simulink subsystem "battery_InputNoise"  (R2022a)
settings: Solver=VariableStepAuto  StartTime=0.0  StopTime=10.0  RelTol=1e-3
values from neighbouring files (symbols this model uses):
  C_des = SIM.OutputMatrix    [RunSimulink.m]
  C_m = C_des(P.cell_voltage,:)    [RunSimulink.m]
  K = -diag(diag_vec)    [getLCParam.m]
  M_cross = LC_param.M_cross    [RunSimulink.m]    (also in getLCParam.m = V*S_cross*U')
  SV_IC = SIM.x_0_FOM    [RunSimulink.m]
  U_NV_NT = LC_param.U_NV_NT    [RunSimulink.m]    (also in getLCParam.m = U_null*V_null')
undefined symbols (not defined in the file or in its folder): AN, CA, CONS, EL, FLAG, N, P, PROPS, SEP, SIM, tc
libraries: simulink x2
settings Model: Creator=tyevans  LastModifiedBy=tyevans

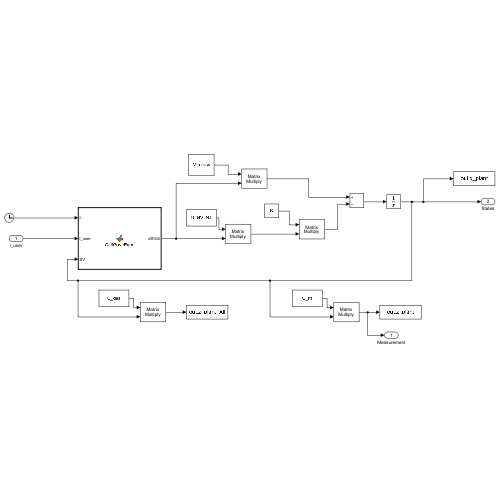
[thumbnail: Simulink's stored preview of the top-level diagram]
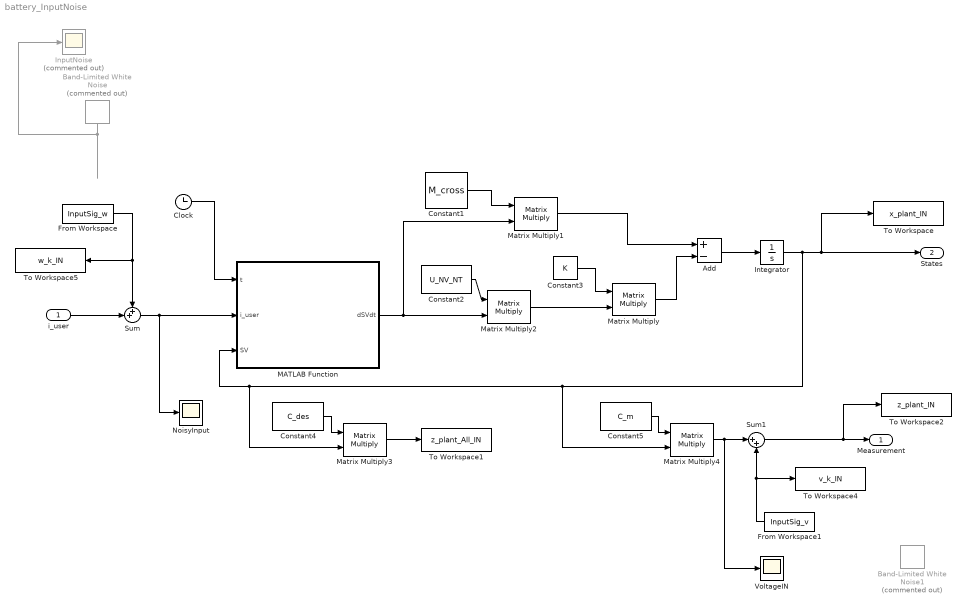
== system battery_InputNoise ==
  i_user : Inport
  Add : Sum  Inputs=+-
  Band-Limited White Noise : simulink/Sources/Band-Limited White Noise  Commented=on  Cov=pow_Qi  Ts=tc  seed=[100]  VectorParams1D=off
  Band-Limited White Noise1 : simulink/Sources/Band-Limited White Noise  Commented=on  Cov=pow_R  Ts=tc  seed=[23341]  VectorParams1D=off
  Clock : Clock
  Constant1 : Constant  Value=M_cross  VectorParams1D=off
  Constant2 : Constant  Value=U_NV_NT  VectorParams1D=off
  Constant3 : Constant  Value=K  VectorParams1D=off
  Constant4 : Constant  Value=C_des  VectorParams1D=off
  Constant5 : Constant  Value=C_m  VectorParams1D=off
  From Workspace : FromWorkspace  VariableName=InputSig_w  OutputAfterFinalValue=Holding final value
  From Workspace1 : FromWorkspace  VariableName=InputSig_v  OutputAfterFinalValue=Holding final value
  InputNoise : Scope  Commented=on
  Integrator : Integrator  InitialCondition=SV_IC
  MATLAB Function : MATLAB Function  TreatAsAtomicUnit=on
  Matrix Multiply{,1..4} (5 alike) : Product  Multiplication=Matrix(*)
  NoisyInput : Scope
  Sum : Sum  Inputs=++|
  Sum1 : Sum  Inputs=|++
  To Workspace : ToWorkspace  VariableName=x_plant_IN  SaveFormat=Structure With Time  SampleTime=-1
  To Workspace1 : ToWorkspace  VariableName=z_plant_All_IN  SaveFormat=Structure With Time  SampleTime=-1
  To Workspace2 : ToWorkspace  VariableName=z_plant_IN  SaveFormat=Structure With Time  SampleTime=-1
  To Workspace4 : ToWorkspace  VariableName=v_k_IN  SaveFormat=Structure With Time  SampleTime=-1
  To Workspace5 : ToWorkspace  VariableName=w_k_IN  SaveFormat=Structure With Time  SampleTime=-1
      settings: Save2DSignal=2-D array (concatenate along first dimension)
  VoltageIN : Scope
  Measurement : Outport
  States : Outport  Port=2
  wires:
  Constant2/1 -> Matrix Multiply2/1
  Matrix Multiply/1 -> Add/2
  Matrix Multiply1/1 -> Add/1
  Clock/1 -> MATLAB Function/1(t)
  Constant3/1 -> Matrix Multiply/1
  Constant4/1 -> Matrix Multiply3/1
  Matrix Multiply3/1 -> To Workspace1/1
  Constant1/1 -> Matrix Multiply1/1
  Add/1 -> Integrator/1
  MATLAB Function/1(dSVdt) -> Matrix Multiply2/2, Matrix Multiply1/2
  Matrix Multiply2/1 -> Matrix Multiply/2
  Constant5/1 -> Matrix Multiply4/1
  Integrator/1 -> States/1, To Workspace/1, Matrix Multiply4/2, Matrix Multiply3/2, MATLAB Function/3(SV)
  From Workspace1/1 -> Sum1/2, To Workspace4/1
  Matrix Multiply4/1 -> Sum1/1, VoltageIN/1
  Sum1/1 -> To Workspace2/1, Measurement/1
  i_user/1 -> Sum/2
  Sum/1 -> MATLAB Function/2(i_user), NoisyInput/1
  Band-Limited White Noise/1 -> InputNoise/1
  From Workspace/1 -> To Workspace5/1, Sum/1

== matlab function battery_InputNoise/MATLAB Function ==
  data: t input; i_user input; dSVdt output; SV input; AN parameter; CA parameter; SEP parameter; EL parameter; SIM parameter; CONS parameter; P parameter; N parameter; FLAG parameter; PROPS parameter
function dSVdt = CallGovnEqns(t,i_user,SV, AN, CA, SEP, EL, SIM, CONS, P, N, FLAG, PROPS)
% Initialize Output
dSVdt = zeros(N.N_SV_tot,1);

% Call GovnEqns
coder.extrinsic('ConvertStrCallGov')
[dSVdt] = ConvertStrCallGov(t,SV,AN,CA,SEP,EL,SIM,CONS,P,N,FLAG,PROPS,i_user);

end
